simulink model "DAQ_and_Motor_Control_Test"  (Simulink 6.6)
settings: Solver=FixedStepDiscrete  StartTime=0.0  StopTime=inf  FixedStep=parameters.model.sample_time  RelTol=1e-3
undefined symbols (not defined in the file or in its folder): parameters
libraries: simulink x2, ni_lib x2
settings Model: Creator=research  LastModifiedBy=research

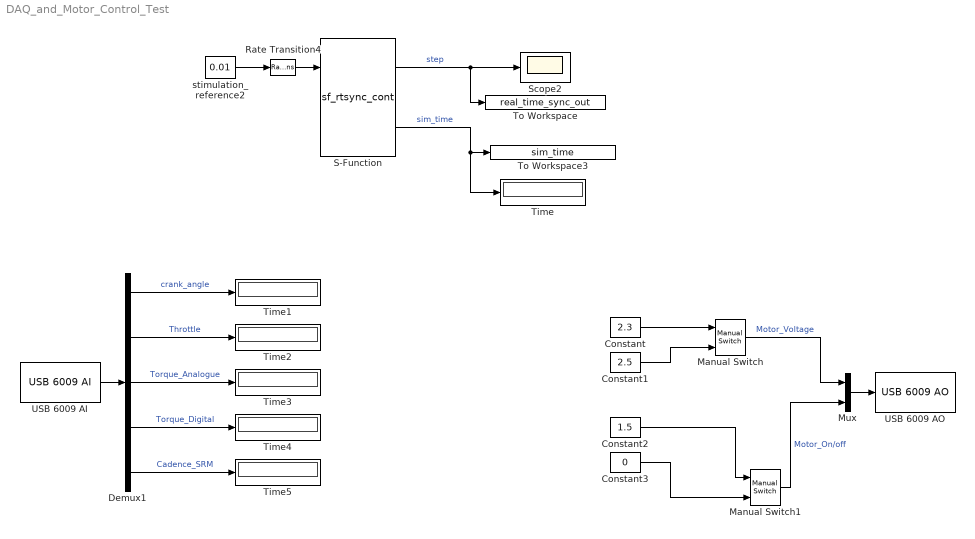
== system DAQ_and_Motor_Control_Test ==
  Constant : Constant  Value=2.3
  Constant1 : Constant  Value=2.5
  Constant2 : Constant  Value=1.5
  Constant3 : Constant  Value=0
  Demux1 : Demux  Outputs=5
  Manual Switch : simulink/Signal Routing/Manual Switch  SystemSampleTime=-1  sw=0  action=0  varsize=off
  Manual Switch1 : simulink/Signal Routing/Manual Switch  SystemSampleTime=-1  sw=0  action=0  varsize=off
  Mux : Mux  Inputs=2
  Rate Transition4 : RateTransition  X0=0.011  OutPortSampleTime=parameters.model.sample_time
  S-Function : S-Function  FunctionName=sf_rtsync_cont  Parameters=1
  Scope2 : Scope
      settings: YMin=-3.46945e-018  YMax=0.12
  Time{,1..5} (6 alike) : Display
  To Workspace : ToWorkspace  VariableName=real_time_sync_out  SampleTime=parameters.model.sample_time  SaveFormat=Array
  To Workspace3 : ToWorkspace  VariableName=sim_time  SampleTime=-1  SaveFormat=Array
      settings: Decimation=5
  USB 6009 AI : ni_lib/USB 6009 AI  channels=[1 2 3 4 5]  Ts=5  inp_min=-5  inp_max=5  terminalcfg=RSE
  USB 6009 AO : ni_lib/USB 6009 AO  channels=[1 2]  Ts=5  inp_min=0  inp_max=5
  stimulation_reference2 : Constant  Value=0.01
      mask Type: text(0.5,0.5,'bla_name.bla', 'VerticalAlignment', 'middle', 'HorizontalAlignment', 'centre')
  wires:
  S-Function/2 -> To Workspace3/1, Time/1  "sim_time"
  S-Function/1 -> Scope2/1, To Workspace/1  "step"
  Rate Transition4/1 -> S-Function/1
  stimulation_reference2/1 -> Rate Transition4/1
  USB 6009 AI/1 -> Demux1/1
  Demux1/1 -> Time1/1  "crank_angle"
  Demux1/2 -> Time2/1  "Throttle"
  Demux1/3 -> Time3/1  "Torque_Analogue"
  Demux1/4 -> Time4/1  "Torque_Digital"
  Demux1/5 -> Time5/1  "Cadence_SRM"
  Mux/1 -> USB 6009 AO/1
  Manual Switch/1 -> Mux/1  "Motor_Voltage"
  Manual Switch1/1 -> Mux/2  "Motor_On/off"
  Constant/1 -> Manual Switch/1
  Constant1/1 -> Manual Switch/2
  Constant2/1 -> Manual Switch1/1
  Constant3/1 -> Manual Switch1/2
